simulink model "simulink_SS1"  (R2020a)
settings: Solver=VariableStepAuto  StartTime=0.0  StopTime=5  RelTol=1e-3
settings Model: Creator=啊包PC  LastModifiedBy=啊包PC

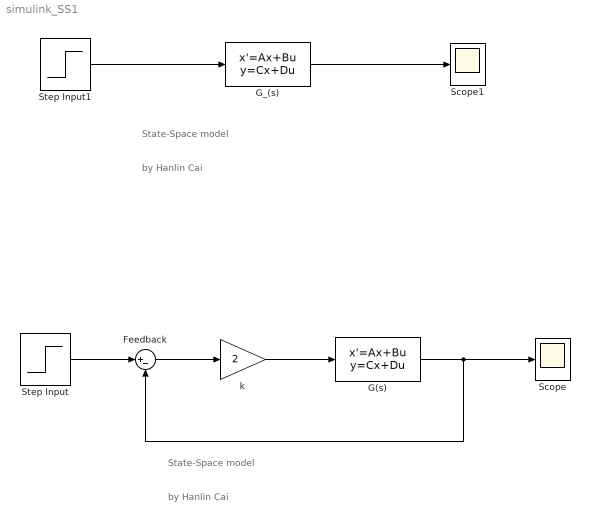
== system simulink_SS1 ==
  note: by Hanlin Cai
  note: State-Space model
  note: State-Space model
  note: by Hanlin Cai
  Feedback : Sum  Inputs=|+-
  G(s) : StateSpace  A=[0 1;-25 -10]  B=[0 ; 1]  C=[-4 4]  D=0  InitialCondition=0
  G_(s) : StateSpace  A=[0 1;-25 -10]  B=[0 ; 1]  C=[-4 4]  D=0  InitialCondition=0
  Scope : Scope
  Scope1 : Scope
  Step Input : Step  Time=0  Before=1000  SampleTime=0
  Step Input1 : Step  Time=0  SampleTime=0
  k : Gain  Gain=2
  wires:
  G(s)/1 -> Feedback/2, Scope/1
  Step Input/1 -> Feedback/1
  Feedback/1 -> k/1
  k/1 -> G(s)/1
  Step Input1/1 -> G_(s)/1
  G_(s)/1 -> Scope1/1
